simulink subsystem "mixer"  (R2026a)
settings: Solver=VariableStepAuto
settings Model: Creator=Kiril  LastModifiedBy=Kiril

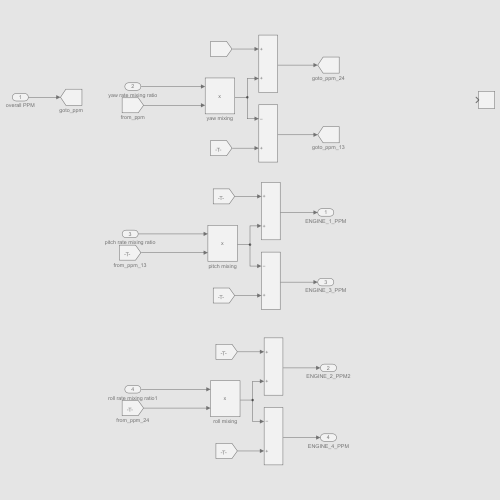
[thumbnail: Simulink's stored preview of the top-level diagram]
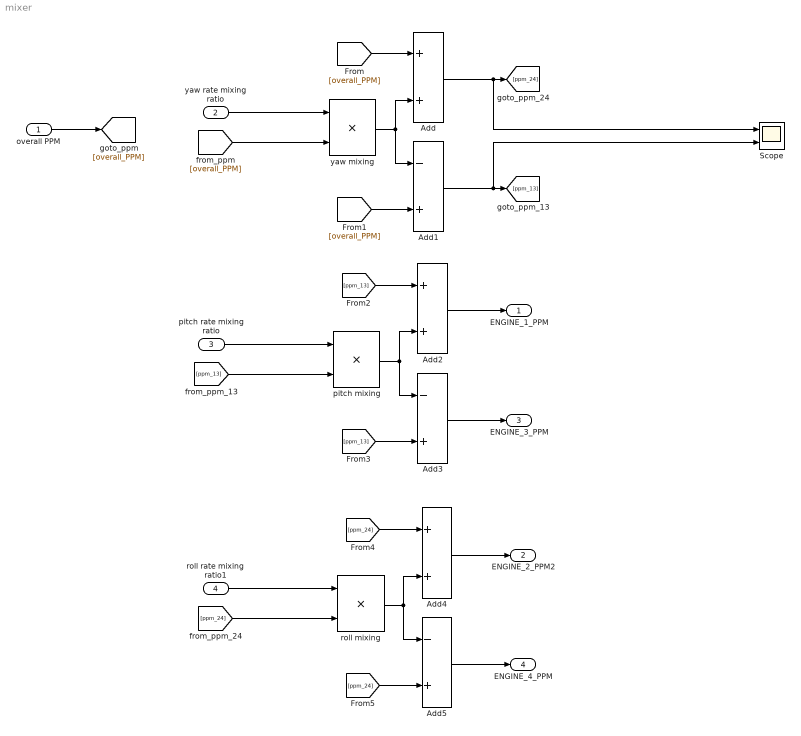
== system mixer ==
  overall PPM : Inport
  yaw rate mixing ratio : Inport  Port=2
  pitch rate mixing ratio : Inport  Port=3
  roll rate mixing ratio1 : Inport  Port=4
  Add : Sum
  Add1 : Sum  Inputs=-+
  Add2 : Sum
  Add3 : Sum  Inputs=-+
  Add4 : Sum
  Add5 : Sum  Inputs=-+
  Scope : Scope  NumInputPorts=2
      settings: ActiveDisplayYMinimum=7.2641558851961463  ActiveDisplayYMaximum=184.50073413616923  DataLoggingVariableName=ScopeData2
  pitch mixing : Product
  roll mixing : Product
  yaw mixing : Product
  ENGINE_1_PPM : Outport
  ENGINE_2_PPM2 : Outport  Port=2
  ENGINE_3_PPM : Outport  Port=3
  ENGINE_4_PPM : Outport  Port=4
  wires:
  yaw rate mixing ratio/1 -> yaw mixing/1
  overall PPM/1 -> [overall_PPM]
  [overall_PPM] -> yaw mixing/2
  [overall_PPM] -> Add/1
  yaw mixing/1 -> Add/2, Add1/1
  [overall_PPM] -> Add1/2
  Add/1 -> [ppm_24], Scope/1
  Add1/1 -> [ppm_13], Scope/2
  pitch rate mixing ratio/1 -> pitch mixing/1
  [ppm_13] -> pitch mixing/2
  Add2/1 -> ENGINE_1_PPM/1
  [ppm_13] -> Add2/1
  Add3/1 -> ENGINE_3_PPM/1
  pitch mixing/1 -> Add2/2, Add3/1
  [ppm_13] -> Add3/2
  Add5/1 -> ENGINE_4_PPM/1
  Add4/1 -> ENGINE_2_PPM2/1
  [ppm_24] -> Add4/1
  [ppm_24] -> Add5/2
  [ppm_24] -> roll mixing/2
  roll mixing/1 -> Add5/1, Add4/2
  roll rate mixing ratio1/1 -> roll mixing/1
